simulink model "Project1"  (R2023b)
settings: Solver=ode1  StartTime=0.0  StopTime=25  FixedStep=0.1  RelTol=1e-3
values from neighbouring files (symbols this model uses):
  A = 4    [P1_demo_code.m]    (also in Project1_Part2.m = A_values(l))
  b = 1    [P1_demo_code.m]    (also in Project1_Part2.m = b_values(k))
  J = 1    [P1_demo_code.m]
  w_0 = 4    [P1_demo_code.m]    (also in Project1_Part2.m = w_0_values(i))
settings Model: Creator=saman  LastModifiedBy=saman

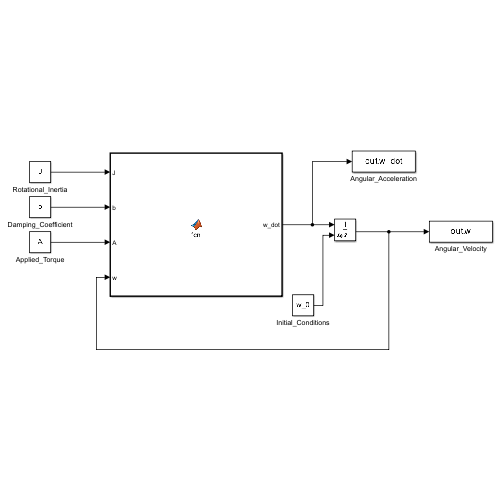
[thumbnail: Simulink's stored preview of the top-level diagram]
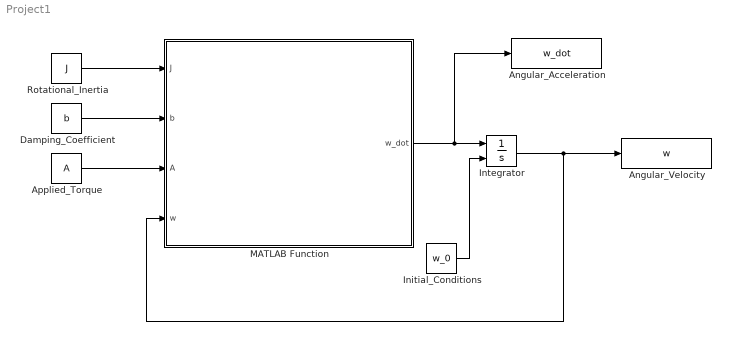
== system Project1 ==
  Angular_Acceleration : ToWorkspace  VariableName=w_dot  SaveFormat=Timeseries  SampleTime=-1
  Angular_Velocity : ToWorkspace  VariableName=w  SaveFormat=Timeseries  SampleTime=-1
  Applied_Torque : Constant  Value=A
  Damping_Coefficient : Constant  Value=b
  Initial_Conditions : Constant  Value=w_0
  Integrator : Integrator  InitialConditionSource=external
  MATLAB Function : MATLAB Function  TreatAsAtomicUnit=on
  Rotational_Inertia : Constant  Value=J
  wires:
  Rotational_Inertia/1 -> MATLAB Function/1(J)
  Damping_Coefficient/1 -> MATLAB Function/2(b)
  Applied_Torque/1 -> MATLAB Function/3(A)
  MATLAB Function/1(w_dot) -> Angular_Acceleration/1, Integrator/1
  Initial_Conditions/1 -> Integrator/2
  Integrator/1 -> Angular_Velocity/1, MATLAB Function/4(w)

== matlab function Project1/MATLAB Function ==
  data: J input; w_dot output; b input; A input; w input
function w_dot = fcn(J, b, A,w)
w_dot = (1/J)*(A-b*w);
end
